simulink model "obiekt_reg"  (R2022b)
settings: Solver=VariableStepAuto  StartTime=0.0  StopTime=20  RelTol=1e-3
undefined symbols (not defined in the file): G, h, y
settings Model: Creator=janro  LastModifiedBy=janro

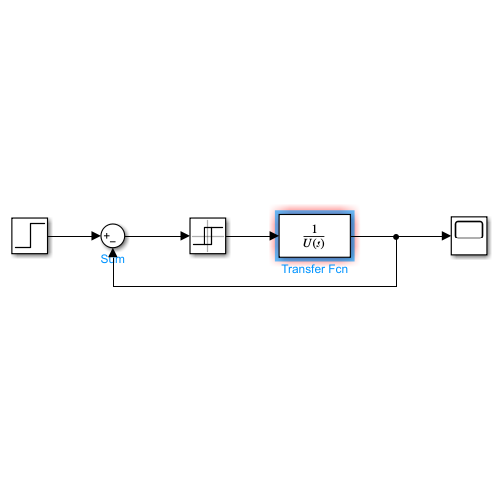
[thumbnail: Simulink's stored preview of the top-level diagram]
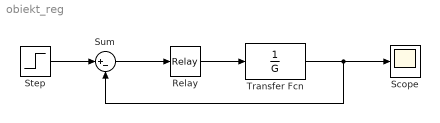
== system obiekt_reg ==
  Relay : Relay  OnSwitchValue=h  OffSwitchValue=-h  OnOutputValue=y  OffOutputValue=-y
  Scope : Scope
  Step : Step  SampleTime=0
  Sum : Sum  Inputs=|+-
  Transfer Fcn : TransferFcn  Denominator=G
  wires:
  Step/1 -> Sum/1
  Sum/1 -> Relay/1
  Relay/1 -> Transfer Fcn/1
  Transfer Fcn/1 -> Sum/2, Scope/1
